simulink model "exampleModel_bus_axi_lcls2"  (R2017b)
settings: Solver=VariableStepAuto  StartTime=0.0  StopTime=10e-5  RelTol=1e-3
PreLoadFcn:
  | setup
values from neighbouring files (symbols this model uses):
  axiClk = 156.25e6    (= 156250000)    [setup.m]    (also in setup_exampleModel_bus_axi_simulink.m; setup_exampleModel_bus_axi_simulink_lcls2.m; setup_lcls2_pcav.m; sysgen_signal.m)
  cav1p1_addr = 204    [setup_exampleModel_bus_axi_simulink.m]    (also in setup_exampleModel_bus_axi_simulink_lcls2.m; setup_lcls2_pcav.m; sysgen_signal.m)
  cav1p2_addr = cav1p1_addr * 2    (= 408)    [setup_exampleModel_bus_axi_simulink.m]    (also in setup_exampleModel_bus_axi_simulink_lcls2.m; setup_lcls2_pcav.m; sysgen_signal.m)
  cav2p1_addr = cav1p1_addr * 3    (= 612)    [setup_exampleModel_bus_axi_simulink.m]    (also in setup_exampleModel_bus_axi_simulink_lcls2.m; setup_lcls2_pcav.m; sysgen_signal.m)
  cav2p2_addr = cav1p1_addr * 4    (= 816)    [setup_exampleModel_bus_axi_simulink.m]    (also in setup_exampleModel_bus_axi_simulink_lcls2.m; setup_lcls2_pcav.m; sysgen_signal.m)
  Fadc = Fs/interleavedChannels    (= 29750000)    [setup.m]    (also in setup_exampleModel_bus_axi_simulink.m = 357000000; setup_exampleModel_bus_axi_simulink_lcls2.m = 351000000; setup_lcls2_pcav.m = 357000000; sysgen_signal.m = 357000000)
  Fproc = 204e6    (= 204000000)    [setup_exampleModel_bus_axi_simulink.m]    (also in setup_exampleModel_bus_axi_simulink_lcls2.m = 200571400; setup_lcls2_pcav.m; sysgen_signal.m)
  Fsig = Fproc/12    (= 17000000)    [setup_exampleModel_bus_axi_simulink.m]    (also in setup_exampleModel_bus_axi_simulink_lcls2.m = 16714283.3333; setup_lcls2_pcav.m)
  Tadc = 1/fadc    (= 2.80112044818e-09)    [cavity_signal.m]    (also in setup_exampleModel_bus_axi_simulink.m; setup_exampleModel_bus_axi_simulink_lcls2.m = 2.849002849e-09; setup_lcls2_pcav.m; setup_pcav_simulink.m)
undefined symbols (not defined in the file or in its folder): AXI4, Lite
libraries: xbsIndex_r4 x2055, llrf_lib x10, simulink x1
(part 8 of 12)

== system exampleModel_bus_axi_lcls2/example/dsp/Cav2/c1p1_Masking_window ==
  note: delay for the comparison because Axilite register
      | takes a about 40 dsp clk cycles to load in
  counter : Inport
  start_pt : Inport  Port=2
  stop_pt : Inport  Port=3
  Constant1 : xbsIndex_r4/Constant  const=0  gui_display_data_type=Fixed-point  arith_type=Unsigned  n_bits=16  bin_pt=0  preci_type=Single  exp_width=8  frac_width=24  explicit_period=off  period=1  equ=P=C  opselect=C  inp2=PCIN>>17  opr=+  inp1=P  carry=CIN  dbl_ovrd=off  block_type=constant
  Convert11 : xbsIndex_r4/Convert  gui_display_data_type=Fixed-point  arith_type=Unsigned  n_bits=1  bin_pt=0  float_type=Single  exp_bits=8  fraction_bits=24  quantization=Truncate  overflow=Wrap  en=off  latency=1  pipeline=off  dbl_ovrd=off  block_type=convert
  Delay{1..4} (4 alike) : xbsIndex_r4/Delay  rst=off  infoeditControl=Selection of Reset will increase slice count due to use of real FFs and instead of SRLs  en=off  latency=1  reg_retiming=off  dbl_ovrd=off  block_type=delay
  Down Sample1 : xbsIndex_r4/Down Sample  sample_ratio=12  sample_phase="Last Value of Frame  (most efficient)"  en=off  rst=off  latency=1  dbl_ovrd=off  block_type=dsamp
  Down Sample2 : xbsIndex_r4/Down Sample  sample_ratio=12  sample_phase="Last Value of Frame  (most efficient)"  en=off  rst=off  latency=1  dbl_ovrd=off  block_type=dsamp
  Logical1 : xbsIndex_r4/Logical  logical_function=AND  inputs=2  en=off  latency=1  precision=Full  arith_type=Unsigned  n_bits=16  bin_pt=0  align_bp=on  dbl_ovrd=off  block_type=logical
  Register5 : xbsIndex_r4/Register  init=0  rst=off  en=off  dbl_ovrd=off  block_type=register
  Register6 : xbsIndex_r4/Register  init=100  rst=off  en=off  dbl_ovrd=off  block_type=register
  Relational2 : xbsIndex_r4/Relational  mode=a>b  op_type=Bool  en=off  latency=1  dbl_ovrd=off  block_type=relational
  Relational3 : xbsIndex_r4/Relational  mode=a<b  op_type=Bool  en=on  latency=1  dbl_ovrd=off  block_type=relational
  Relational4 : xbsIndex_r4/Relational  mode=a>b  op_type=Bool  en=on  latency=1  dbl_ovrd=off  block_type=relational
  eval_window : Outport
  wires:
  start_pt/1 -> Register5/1
  Register5/1 -> Down Sample1/1
  stop_pt/1 -> Register6/1
  Register6/1 -> Down Sample2/1
  Delay2/1 -> Relational4/2
  Delay3/1 -> [stop], Relational3/2
  Constant1/1 -> Relational2/2
  Logical1/1 -> Convert11/1
  Relational3/1 -> Logical1/2
  Convert11/1 -> eval_window/1
  Relational2/1 -> [enb], Relational3/3, Relational4/3
  counter/1 -> [cntr]
  Down Sample1/1 -> Delay2/1
  Down Sample2/1 -> Delay3/1
  Delay1/1 -> Relational4/1
  Delay4/1 -> Relational3/1
  Relational4/1 -> Logical1/1
  [cntr] -> Relational2/1, Delay1/1, Delay4/1

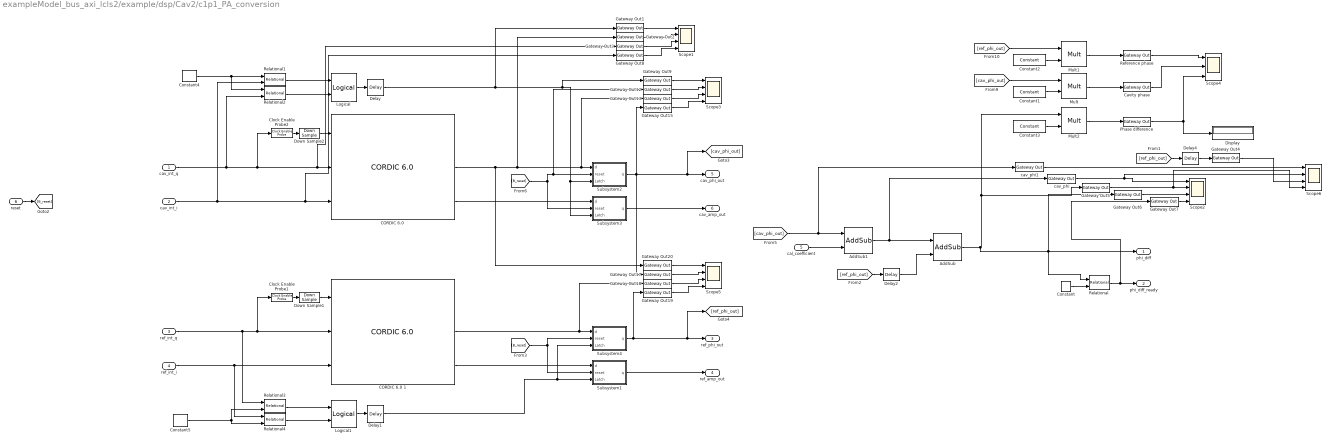
== system exampleModel_bus_axi_lcls2/example/dsp/Cav2/c1p1_PA_conversion ==
  cav_int_q : Inport
  cav_int_i : Inport  Port=2
  ref_int_q : Inport  Port=3
  ref_int_i : Inport  Port=4
  cal_coefficient : Inport  Port=5
  reset : Inport  Port=6
  AddSub : xbsIndex_r4/AddSub  mode=Subtraction  use_carryin=off  use_carryout=off  en=off  latency=1  precision=User Defined  arith_type="Signed  (2's comp)"  n_bits=18  bin_pt=15  quantization=Truncate  overflow=Wrap  use_behavioral_HDL=off  hw_selection=Fabric  pipelined=off  dbl_ovrd=off  block_type=addsub
  AddSub1 : xbsIndex_r4/AddSub  mode=Addition  use_carryin=off  use_carryout=off  en=off  latency=1  precision=User Defined  arith_type="Signed  (2's comp)"  n_bits=18  bin_pt=15  quantization=Truncate  overflow=Wrap  use_behavioral_HDL=off  hw_selection=Fabric  pipelined=off  dbl_ovrd=off  block_type=addsub
  "CORDIC 6.0 " : xbsIndex_r4/CORDIC 6.0   functional_selection=Translate  architectural_configuration=Parallel  pipelining_mode=Maximum  data_format=SignedFraction  phase_format=Scaled_Radians  input_width=18  output_width=18  round_mode=Truncate  iterations=0  precision=0  compensation_scaling=No_Scale_Compensation  coarse_rotation=on  aclken=off  aresetn=off  out_tready=off  cartesian_has_tuser=off  cartesian_has_tlast=off  cartesian_tuser_width=1  phase_has_tuser=off  phase_has_tlast=off  phase_tuser_width=1  out_tlast_behv=Null  flow_control=NonBlocking  optimize_goal=Resources  trim_axipin_name=on  simulation_type=hybrid_sim  simulation_model=sysgen:cordic_v6_0  data_path_portlist={'s_axis_cartesian_tdata_imag', 's_axis_cartesian_tdata_real', 's_axis_phase_tdata_phase', 'm_axis_dout_tdata_imag', 'm_axis_dout_tdata_real', 'm_axis_dout_tdata_phase','m_axis_dout_tdata'}  ip_name=CORDIC  ip_version=6.0  dsptool_ready=true  ipcore_usecache=true  ipcore_useipmodelcache=true  wrapper_available=true  port_translation_map={ 'aclken' => 'en', 'aresetn' => 'rst' }  block_type=cordic_v6_0
      settings: infoedit=CORDIC 6.0
  CORDIC 6.0 1 : xbsIndex_r4/CORDIC 6.0   functional_selection=Translate  architectural_configuration=Parallel  pipelining_mode=Maximum  data_format=SignedFraction  phase_format=Scaled_Radians  input_width=18  output_width=18  round_mode=Truncate  iterations=0  precision=0  compensation_scaling=No_Scale_Compensation  coarse_rotation=on  aclken=off  aresetn=off  out_tready=off  cartesian_has_tuser=off  cartesian_has_tlast=off  cartesian_tuser_width=1  phase_has_tuser=off  phase_has_tlast=off  phase_tuser_width=1  out_tlast_behv=Null  flow_control=NonBlocking  optimize_goal=Resources  trim_axipin_name=on  simulation_type=hybrid_sim  simulation_model=sysgen:cordic_v6_0  data_path_portlist={'s_axis_cartesian_tdata_imag', 's_axis_cartesian_tdata_real', 's_axis_phase_tdata_phase', 'm_axis_dout_tdata_imag', 'm_axis_dout_tdata_real', 'm_axis_dout_tdata_phase','m_axis_dout_tdata'}  ip_name=CORDIC  ip_version=6.0  dsptool_ready=true  ipcore_usecache=true  ipcore_useipmodelcache=true  wrapper_available=true  port_translation_map={ 'aclken' => 'en', 'aresetn' => 'rst' }  block_type=cordic_v6_0
      settings: infoedit=CORDIC 6.0
  Cavity phase : xbsIndex_r4/Gateway Out  inherit_from_input=off  hdl_port=off  rows=1  columns=1  UseAsDAC=off  DACChannel='1'  interface=None  automatic_assignment=on  address_offset=hex2dec('00')  intf_name=''  intf_description=''  timing_constraint=None  locs_specified=off  LOCs={}  io_standard={}  block_type=gatewayout
  Clock Enable Probe1 : xbsIndex_r4/Clock Enable Probe  inherit_constraints=on  block_type=ceprobe
      settings: infoedit="Clock enable extractor.  Produces a Boolean output that mirrors the hardware clock enable associated with the input sample rate.<br><br>Hardware notes: in hardware this block costs nothing."
  Clock Enable Probe2 : xbsIndex_r4/Clock Enable Probe  inherit_constraints=on  block_type=ceprobe
      settings: infoedit="Clock enable extractor.  Produces a Boolean output that mirrors the hardware clock enable associated with the input sample rate.<br><br>Hardware notes: in hardware this block costs nothing."
  Constant : xbsIndex_r4/Constant  const=0  gui_display_data_type=Fixed-point  arith_type=Signed (2's comp)  n_bits=1  bin_pt=0  preci_type=Single  exp_width=8  frac_width=24  explicit_period=off  period=1  equ=P=C  opselect=C  inp2=PCIN>>17  opr=+  inp1=P  carry=CIN  dbl_ovrd=off  block_type=constant
  Constant1 : xbsIndex_r4/Constant  const=pi  gui_display_data_type=Fixed-point  arith_type=Unsigned  n_bits=16  bin_pt=14  preci_type=Single  exp_width=8  frac_width=24  explicit_period=off  period=1  equ=P=C  opselect=C  inp2=PCIN>>17  opr=+  inp1=P  carry=CIN  dbl_ovrd=off  block_type=constant
  Constant2 : xbsIndex_r4/Constant  const=pi  gui_display_data_type=Fixed-point  arith_type=Unsigned  n_bits=16  bin_pt=14  preci_type=Single  exp_width=8  frac_width=24  explicit_period=off  period=1  equ=P=C  opselect=C  inp2=PCIN>>17  opr=+  inp1=P  carry=CIN  dbl_ovrd=off  block_type=constant
  Constant3 : xbsIndex_r4/Constant  const=pi  gui_display_data_type=Fixed-point  arith_type=Unsigned  n_bits=16  bin_pt=14  preci_type=Single  exp_width=8  frac_width=24  explicit_period=off  period=1  equ=P=C  opselect=C  inp2=PCIN>>17  opr=+  inp1=P  carry=CIN  dbl_ovrd=off  block_type=constant
  Constant4 : xbsIndex_r4/Constant  const=0  gui_display_data_type=Fixed-point  arith_type=Signed (2's comp)  n_bits=16  bin_pt=14  preci_type=Single  exp_width=8  frac_width=24  explicit_period=off  period=1  equ=P=C  opselect=C  inp2=PCIN>>17  opr=+  inp1=P  carry=CIN  dbl_ovrd=off  block_type=constant
  Constant5 : xbsIndex_r4/Constant  const=0  gui_display_data_type=Fixed-point  arith_type=Signed (2's comp)  n_bits=16  bin_pt=14  preci_type=Single  exp_width=8  frac_width=24  explicit_period=off  period=1  equ=P=C  opselect=C  inp2=PCIN>>17  opr=+  inp1=P  carry=CIN  dbl_ovrd=off  block_type=constant
  Delay : xbsIndex_r4/Delay  rst=off  infoeditControl=Selection of Reset will increase slice count due to use of real FFs and instead of SRLs  en=off  latency=21  reg_retiming=off  dbl_ovrd=off  block_type=delay
  Delay1 : xbsIndex_r4/Delay  rst=off  infoeditControl=Selection of Reset will increase slice count due to use of real FFs and instead of SRLs  en=off  latency=21  reg_retiming=off  dbl_ovrd=off  block_type=delay
  Delay2 : xbsIndex_r4/Delay  rst=off  infoeditControl=Selection of Reset will increase slice count due to use of real FFs and instead of SRLs  en=off  latency=1  reg_retiming=off  dbl_ovrd=off  block_type=delay
  Delay4 : xbsIndex_r4/Delay  rst=off  infoeditControl=Selection of Reset will increase slice count due to use of real FFs and instead of SRLs  en=off  latency=1  reg_retiming=off  dbl_ovrd=off  block_type=delay
  Display : Display
  Down Sample1 : xbsIndex_r4/Down Sample  sample_ratio=12  sample_phase="Last Value of Frame  (most efficient)"  en=off  rst=off  latency=1  dbl_ovrd=off  block_type=dsamp
  Down Sample2 : xbsIndex_r4/Down Sample  sample_ratio=12  sample_phase="Last Value of Frame  (most efficient)"  en=off  rst=off  latency=1  dbl_ovrd=off  block_type=dsamp
  Gateway Out{1..9,12..13,15,17..20} (16 alike) : xbsIndex_r4/Gateway Out  inherit_from_input=off  hdl_port=off  rows=1  columns=1  UseAsDAC=off  DACChannel='1'  interface=None  automatic_assignment=on  address_offset=hex2dec('00')  intf_name=''  intf_description=''  timing_constraint=None  locs_specified=off  LOCs={}  io_standard={}  block_type=gatewayout
  Logical : xbsIndex_r4/Logical  logical_function=AND  inputs=2  en=off  latency=1  precision=Full  arith_type=Unsigned  n_bits=16  bin_pt=0  align_bp=on  dbl_ovrd=off  block_type=logical
  Logical1 : xbsIndex_r4/Logical  logical_function=AND  inputs=2  en=off  latency=1  precision=Full  arith_type=Unsigned  n_bits=16  bin_pt=0  align_bp=on  dbl_ovrd=off  block_type=logical
  Mult : xbsIndex_r4/Mult  precision=Full  arith_type="Signed  (2's comp)"  n_bits=16  bin_pt=14  quantization=Truncate  overflow=Wrap  en=off  latency=3  use_behavioral_HDL=off  opt=Speed  use_embedded=on  optimum_pipeline=off  pipeline=on  dbl_ovrd=off  use_rpm=on  placement_style=Triangular  block_type=mult
  Mult1 : xbsIndex_r4/Mult  precision=Full  arith_type="Signed  (2's comp)"  n_bits=16  bin_pt=14  quantization=Truncate  overflow=Wrap  en=off  latency=3  use_behavioral_HDL=off  opt=Speed  use_embedded=on  optimum_pipeline=off  pipeline=on  dbl_ovrd=off  use_rpm=on  placement_style=Triangular  block_type=mult
  Mult2 : xbsIndex_r4/Mult  precision=Full  arith_type="Signed  (2's comp)"  n_bits=16  bin_pt=14  quantization=Truncate  overflow=Wrap  en=off  latency=3  use_behavioral_HDL=off  opt=Speed  use_embedded=on  optimum_pipeline=off  pipeline=on  dbl_ovrd=off  use_rpm=on  placement_style=Triangular  block_type=mult
  Phase difference : xbsIndex_r4/Gateway Out  inherit_from_input=off  hdl_port=off  rows=1  columns=1  UseAsDAC=off  DACChannel='1'  interface=None  automatic_assignment=on  address_offset=hex2dec('00')  intf_name=''  intf_description=''  timing_constraint=None  locs_specified=off  LOCs={}  io_standard={}  block_type=gatewayout
  Reference phase : xbsIndex_r4/Gateway Out  inherit_from_input=off  hdl_port=off  rows=1  columns=1  UseAsDAC=off  DACChannel='1'  interface=None  automatic_assignment=on  address_offset=hex2dec('00')  intf_name=''  intf_description=''  timing_constraint=None  locs_specified=off  LOCs={}  io_standard={}  block_type=gatewayout
  Relational{,1..4} (5 alike) : xbsIndex_r4/Relational  mode=a!=b  op_type=Bool  en=off  latency=1  dbl_ovrd=off  block_type=relational
  Scope{1..3,5..6} (5 alike) : Scope  NumInputPorts=4
  Scope4 : Scope  NumInputPorts=3
  Subsystem1 : Subsystem
  Subsystem2 : Subsystem
  Subsystem3 : Subsystem
  Subsystem4 : Subsystem
  cav_phi : xbsIndex_r4/Gateway Out  inherit_from_input=off  hdl_port=off  rows=1  columns=1  UseAsDAC=off  DACChannel='1'  interface=None  automatic_assignment=on  address_offset=hex2dec('00')  intf_name=''  intf_description=''  timing_constraint=None  locs_specified=off  LOCs={}  io_standard={}  block_type=gatewayout
  cav_phi1 : xbsIndex_r4/Gateway Out  inherit_from_input=off  hdl_port=off  rows=1  columns=1  UseAsDAC=off  DACChannel='1'  interface=None  automatic_assignment=on  address_offset=hex2dec('00')  intf_name=''  intf_description=''  timing_constraint=None  locs_specified=off  LOCs={}  io_standard={}  block_type=gatewayout
  phi_diff : Outport
  phi_diff_ready : Outport  Port=2
  ref_phi_out : Outport  Port=3
  ref_amp_out : Outport  Port=4
  cav_phi_out : Outport  Port=5
  cav_amp_out : Outport  Port=6
  wires:
  ref_int_i/1 -> CORDIC 6.0 1/3, Relational4/1
  ref_int_q/1 -> Relational3/1, CORDIC 6.0 1/2, Clock Enable Probe1/1
  [ref_phi_out] -> Delay4/1
  AddSub1/1 -> cav_phi/1, AddSub/1
  [cav_phi_out] -> cav_phi1/1, AddSub1/1
  cal_coefficient/1 -> AddSub1/2
  Subsystem4/1(q) -> Gateway Out19/1, [ref_phi_out], ref_phi_out/1
  Subsystem1/1(q) -> ref_amp_out/1
  Subsystem2/1(q) -> Gateway Out17/1, Gateway Out15/1, [cav_phi_out], cav_phi_out/1
  Subsystem3/1(q) -> cav_amp_out/1
  reset/1 -> [B_reset]
  [B_reset] -> Subsystem4/2(reset), Subsystem1/2(reset)
  [B_reset] -> Subsystem3/2(reset), Gateway Out12/1, Subsystem2/2(reset)
  AddSub/1 -> Gateway Out6/1, phi_diff/1, Relational/1, Mult2/1, Gateway Out5/1
  Delay2/1 -> AddSub/2
  Gateway Out5/1 -> Scope6/4, Scope2/2
  cav_phi/1 -> Scope6/2, Scope2/1
  Gateway Out6/1 -> Scope2/3
  Gateway Out7/1 -> Scope2/4
  Constant/1 -> Relational/2
  Relational/1 -> Gateway Out7/1, phi_diff_ready/1
  Constant1/1 -> Mult/2
  [cav_phi_out] -> Mult/1
  [ref_phi_out] -> Mult1/1
  Constant2/1 -> Mult1/2
  Mult1/1 -> Reference phase/1
  Mult/1 -> Cavity phase/1
  Mult2/1 -> Phase difference/1
  Constant3/1 -> Mult2/2
  Cavity phase/1 -> Scope4/2
  Reference phase/1 -> Scope4/1
  Phase difference/1 -> Display/1, Scope4/3
  Clock Enable Probe2/1 -> Down Sample2/1
  Down Sample2/1 -> "CORDIC 6.0 "/1
  cav_int_q/1 -> Relational2/2, Clock Enable Probe2/1, Gateway Out3/1, "CORDIC 6.0 "/2
  Logical/1 -> Delay/1
  Relational2/1 -> Logical/2
  Relational1/1 -> Logical/1
  cav_int_i/1 -> Relational1/2, Gateway Out8/1, "CORDIC 6.0 "/3
  Constant4/1 -> Relational2/1, Relational1/1
  Delay/1 -> Gateway Out1/1, Gateway Out9/1, Subsystem3/3(Latch), Subsystem2/3(Latch)
  Clock Enable Probe1/1 -> Down Sample1/1
  Down Sample1/1 -> CORDIC 6.0 1/1
  Delay1/1 -> Subsystem4/3(Latch), Subsystem1/3(Latch)
  Relational3/1 -> Logical1/1
  Relational4/1 -> Logical1/2
  Logical1/1 -> Delay1/1
  Constant5/1 -> Relational4/2, Relational3/2
  CORDIC 6.0 1/3 -> Subsystem1/1(d)
  CORDIC 6.0 1/2 -> Gateway Out18/1, Subsystem4/1(d)
  "CORDIC 6.0 "/2 -> Gateway Out20/1, Gateway Out2/1, Gateway Out13/1, Subsystem2/1(d)
  "CORDIC 6.0 "/3 -> Subsystem3/1(d)
  Gateway Out8/1 -> Scope1/4
  Gateway Out3/1 -> Scope1/3
  Gateway Out1/1 -> Scope1/1
  Gateway Out2/1 -> Scope1/2
  Gateway Out12/1 -> Scope3/2
  Gateway Out9/1 -> Scope3/1
  Gateway Out13/1 -> Scope3/3
  Gateway Out15/1 -> Scope3/4
  Gateway Out19/1 -> Scope5/4
  Gateway Out18/1 -> Scope5/3
  Gateway Out20/1 -> Scope5/1
  Gateway Out17/1 -> Scope5/2
  cav_phi1/1 -> Scope6/1
  Delay4/1 -> Gateway Out4/1
  Gateway Out4/1 -> Scope6/3
  [ref_phi_out] -> Delay2/1

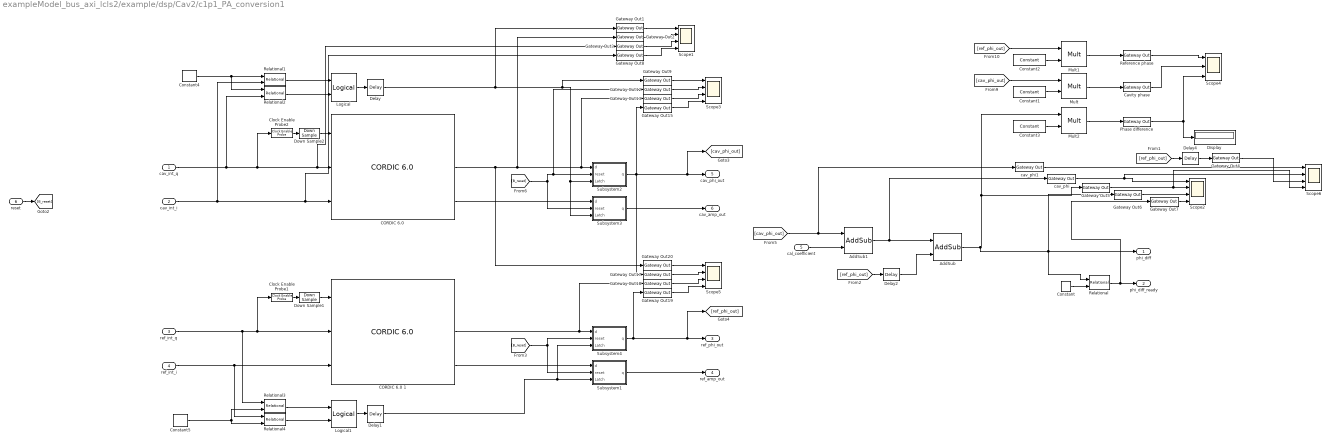
== system exampleModel_bus_axi_lcls2/example/dsp/Cav2/c1p1_PA_conversion1 ==
  cav_int_q : Inport
  cav_int_i : Inport  Port=2
  ref_int_q : Inport  Port=3
  ref_int_i : Inport  Port=4
  cal_coefficient : Inport  Port=5
  reset : Inport  Port=6
  AddSub : xbsIndex_r4/AddSub  mode=Subtraction  use_carryin=off  use_carryout=off  en=off  latency=1  precision=User Defined  arith_type="Signed  (2's comp)"  n_bits=18  bin_pt=15  quantization=Truncate  overflow=Wrap  use_behavioral_HDL=off  hw_selection=Fabric  pipelined=off  dbl_ovrd=off  block_type=addsub
  AddSub1 : xbsIndex_r4/AddSub  mode=Addition  use_carryin=off  use_carryout=off  en=off  latency=1  precision=User Defined  arith_type="Signed  (2's comp)"  n_bits=18  bin_pt=15  quantization=Truncate  overflow=Wrap  use_behavioral_HDL=off  hw_selection=Fabric  pipelined=off  dbl_ovrd=off  block_type=addsub
  "CORDIC 6.0 " : xbsIndex_r4/CORDIC 6.0   functional_selection=Translate  architectural_configuration=Parallel  pipelining_mode=Maximum  data_format=SignedFraction  phase_format=Scaled_Radians  input_width=18  output_width=18  round_mode=Truncate  iterations=0  precision=0  compensation_scaling=No_Scale_Compensation  coarse_rotation=on  aclken=off  aresetn=off  out_tready=off  cartesian_has_tuser=off  cartesian_has_tlast=off  cartesian_tuser_width=1  phase_has_tuser=off  phase_has_tlast=off  phase_tuser_width=1  out_tlast_behv=Null  flow_control=NonBlocking  optimize_goal=Resources  trim_axipin_name=on  simulation_type=hybrid_sim  simulation_model=sysgen:cordic_v6_0  data_path_portlist={'s_axis_cartesian_tdata_imag', 's_axis_cartesian_tdata_real', 's_axis_phase_tdata_phase', 'm_axis_dout_tdata_imag', 'm_axis_dout_tdata_real', 'm_axis_dout_tdata_phase','m_axis_dout_tdata'}  ip_name=CORDIC  ip_version=6.0  dsptool_ready=true  ipcore_usecache=true  ipcore_useipmodelcache=true  wrapper_available=true  port_translation_map={ 'aclken' => 'en', 'aresetn' => 'rst' }  block_type=cordic_v6_0
      settings: infoedit=CORDIC 6.0
  CORDIC 6.0 1 : xbsIndex_r4/CORDIC 6.0   functional_selection=Translate  architectural_configuration=Parallel  pipelining_mode=Maximum  data_format=SignedFraction  phase_format=Scaled_Radians  input_width=18  output_width=18  round_mode=Truncate  iterations=0  precision=0  compensation_scaling=No_Scale_Compensation  coarse_rotation=on  aclken=off  aresetn=off  out_tready=off  cartesian_has_tuser=off  cartesian_has_tlast=off  cartesian_tuser_width=1  phase_has_tuser=off  phase_has_tlast=off  phase_tuser_width=1  out_tlast_behv=Null  flow_control=NonBlocking  optimize_goal=Resources  trim_axipin_name=on  simulation_type=hybrid_sim  simulation_model=sysgen:cordic_v6_0  data_path_portlist={'s_axis_cartesian_tdata_imag', 's_axis_cartesian_tdata_real', 's_axis_phase_tdata_phase', 'm_axis_dout_tdata_imag', 'm_axis_dout_tdata_real', 'm_axis_dout_tdata_phase','m_axis_dout_tdata'}  ip_name=CORDIC  ip_version=6.0  dsptool_ready=true  ipcore_usecache=true  ipcore_useipmodelcache=true  wrapper_available=true  port_translation_map={ 'aclken' => 'en', 'aresetn' => 'rst' }  block_type=cordic_v6_0
      settings: infoedit=CORDIC 6.0
  Cavity phase : xbsIndex_r4/Gateway Out  inherit_from_input=off  hdl_port=off  rows=1  columns=1  UseAsDAC=off  DACChannel='1'  interface=None  automatic_assignment=on  address_offset=hex2dec('00')  intf_name=''  intf_description=''  timing_constraint=None  locs_specified=off  LOCs={}  io_standard={}  block_type=gatewayout
  Clock Enable Probe1 : xbsIndex_r4/Clock Enable Probe  inherit_constraints=on  block_type=ceprobe
      settings: infoedit="Clock enable extractor.  Produces a Boolean output that mirrors the hardware clock enable associated with the input sample rate.<br><br>Hardware notes: in hardware this block costs nothing."
  Clock Enable Probe2 : xbsIndex_r4/Clock Enable Probe  inherit_constraints=on  block_type=ceprobe
      settings: infoedit="Clock enable extractor.  Produces a Boolean output that mirrors the hardware clock enable associated with the input sample rate.<br><br>Hardware notes: in hardware this block costs nothing."
  Constant : xbsIndex_r4/Constant  const=0  gui_display_data_type=Fixed-point  arith_type=Signed (2's comp)  n_bits=1  bin_pt=0  preci_type=Single  exp_width=8  frac_width=24  explicit_period=off  period=1  equ=P=C  opselect=C  inp2=PCIN>>17  opr=+  inp1=P  carry=CIN  dbl_ovrd=off  block_type=constant
  Constant1 : xbsIndex_r4/Constant  const=pi  gui_display_data_type=Fixed-point  arith_type=Unsigned  n_bits=16  bin_pt=14  preci_type=Single  exp_width=8  frac_width=24  explicit_period=off  period=1  equ=P=C  opselect=C  inp2=PCIN>>17  opr=+  inp1=P  carry=CIN  dbl_ovrd=off  block_type=constant
  Constant2 : xbsIndex_r4/Constant  const=pi  gui_display_data_type=Fixed-point  arith_type=Unsigned  n_bits=16  bin_pt=14  preci_type=Single  exp_width=8  frac_width=24  explicit_period=off  period=1  equ=P=C  opselect=C  inp2=PCIN>>17  opr=+  inp1=P  carry=CIN  dbl_ovrd=off  block_type=constant
  Constant3 : xbsIndex_r4/Constant  const=pi  gui_display_data_type=Fixed-point  arith_type=Unsigned  n_bits=16  bin_pt=14  preci_type=Single  exp_width=8  frac_width=24  explicit_period=off  period=1  equ=P=C  opselect=C  inp2=PCIN>>17  opr=+  inp1=P  carry=CIN  dbl_ovrd=off  block_type=constant
  Constant4 : xbsIndex_r4/Constant  const=0  gui_display_data_type=Fixed-point  arith_type=Signed (2's comp)  n_bits=16  bin_pt=14  preci_type=Single  exp_width=8  frac_width=24  explicit_period=off  period=1  equ=P=C  opselect=C  inp2=PCIN>>17  opr=+  inp1=P  carry=CIN  dbl_ovrd=off  block_type=constant
  Constant5 : xbsIndex_r4/Constant  const=0  gui_display_data_type=Fixed-point  arith_type=Signed (2's comp)  n_bits=16  bin_pt=14  preci_type=Single  exp_width=8  frac_width=24  explicit_period=off  period=1  equ=P=C  opselect=C  inp2=PCIN>>17  opr=+  inp1=P  carry=CIN  dbl_ovrd=off  block_type=constant
  Delay : xbsIndex_r4/Delay  rst=off  infoeditControl=Selection of Reset will increase slice count due to use of real FFs and instead of SRLs  en=off  latency=21  reg_retiming=off  dbl_ovrd=off  block_type=delay
  Delay1 : xbsIndex_r4/Delay  rst=off  infoeditControl=Selection of Reset will increase slice count due to use of real FFs and instead of SRLs  en=off  latency=21  reg_retiming=off  dbl_ovrd=off  block_type=delay
  Delay2 : xbsIndex_r4/Delay  rst=off  infoeditControl=Selection of Reset will increase slice count due to use of real FFs and instead of SRLs  en=off  latency=1  reg_retiming=off  dbl_ovrd=off  block_type=delay
  Delay4 : xbsIndex_r4/Delay  rst=off  infoeditControl=Selection of Reset will increase slice count due to use of real FFs and instead of SRLs  en=off  latency=1  reg_retiming=off  dbl_ovrd=off  block_type=delay
  Display : Display
  Down Sample1 : xbsIndex_r4/Down Sample  sample_ratio=12  sample_phase="Last Value of Frame  (most efficient)"  en=off  rst=off  latency=1  dbl_ovrd=off  block_type=dsamp
  Down Sample2 : xbsIndex_r4/Down Sample  sample_ratio=12  sample_phase="Last Value of Frame  (most efficient)"  en=off  rst=off  latency=1  dbl_ovrd=off  block_type=dsamp
  Gateway Out{1..9,12..13,15,17..20} (16 alike) : xbsIndex_r4/Gateway Out  inherit_from_input=off  hdl_port=off  rows=1  columns=1  UseAsDAC=off  DACChannel='1'  interface=None  automatic_assignment=on  address_offset=hex2dec('00')  intf_name=''  intf_description=''  timing_constraint=None  locs_specified=off  LOCs={}  io_standard={}  block_type=gatewayout
  Logical : xbsIndex_r4/Logical  logical_function=AND  inputs=2  en=off  latency=1  precision=Full  arith_type=Unsigned  n_bits=16  bin_pt=0  align_bp=on  dbl_ovrd=off  block_type=logical
  Logical1 : xbsIndex_r4/Logical  logical_function=AND  inputs=2  en=off  latency=1  precision=Full  arith_type=Unsigned  n_bits=16  bin_pt=0  align_bp=on  dbl_ovrd=off  block_type=logical
  Mult : xbsIndex_r4/Mult  precision=Full  arith_type="Signed  (2's comp)"  n_bits=16  bin_pt=14  quantization=Truncate  overflow=Wrap  en=off  latency=3  use_behavioral_HDL=off  opt=Speed  use_embedded=on  optimum_pipeline=off  pipeline=on  dbl_ovrd=off  use_rpm=on  placement_style=Triangular  block_type=mult
  Mult1 : xbsIndex_r4/Mult  precision=Full  arith_type="Signed  (2's comp)"  n_bits=16  bin_pt=14  quantization=Truncate  overflow=Wrap  en=off  latency=3  use_behavioral_HDL=off  opt=Speed  use_embedded=on  optimum_pipeline=off  pipeline=on  dbl_ovrd=off  use_rpm=on  placement_style=Triangular  block_type=mult
  Mult2 : xbsIndex_r4/Mult  precision=Full  arith_type="Signed  (2's comp)"  n_bits=16  bin_pt=14  quantization=Truncate  overflow=Wrap  en=off  latency=3  use_behavioral_HDL=off  opt=Speed  use_embedded=on  optimum_pipeline=off  pipeline=on  dbl_ovrd=off  use_rpm=on  placement_style=Triangular  block_type=mult
  Phase difference : xbsIndex_r4/Gateway Out  inherit_from_input=off  hdl_port=off  rows=1  columns=1  UseAsDAC=off  DACChannel='1'  interface=None  automatic_assignment=on  address_offset=hex2dec('00')  intf_name=''  intf_description=''  timing_constraint=None  locs_specified=off  LOCs={}  io_standard={}  block_type=gatewayout
  Reference phase : xbsIndex_r4/Gateway Out  inherit_from_input=off  hdl_port=off  rows=1  columns=1  UseAsDAC=off  DACChannel='1'  interface=None  automatic_assignment=on  address_offset=hex2dec('00')  intf_name=''  intf_description=''  timing_constraint=None  locs_specified=off  LOCs={}  io_standard={}  block_type=gatewayout
  Relational{,1..4} (5 alike) : xbsIndex_r4/Relational  mode=a!=b  op_type=Bool  en=off  latency=1  dbl_ovrd=off  block_type=relational
  Scope{1..3,5..6} (5 alike) : Scope  NumInputPorts=4
  Scope4 : Scope  NumInputPorts=3
  Subsystem1 : Subsystem
  Subsystem2 : Subsystem
  Subsystem3 : Subsystem
  Subsystem4 : Subsystem
  cav_phi : xbsIndex_r4/Gateway Out  inherit_from_input=off  hdl_port=off  rows=1  columns=1  UseAsDAC=off  DACChannel='1'  interface=None  automatic_assignment=on  address_offset=hex2dec('00')  intf_name=''  intf_description=''  timing_constraint=None  locs_specified=off  LOCs={}  io_standard={}  block_type=gatewayout
  cav_phi1 : xbsIndex_r4/Gateway Out  inherit_from_input=off  hdl_port=off  rows=1  columns=1  UseAsDAC=off  DACChannel='1'  interface=None  automatic_assignment=on  address_offset=hex2dec('00')  intf_name=''  intf_description=''  timing_constraint=None  locs_specified=off  LOCs={}  io_standard={}  block_type=gatewayout
  phi_diff : Outport
  phi_diff_ready : Outport  Port=2
  ref_phi_out : Outport  Port=3
  ref_amp_out : Outport  Port=4
  cav_phi_out : Outport  Port=5
  cav_amp_out : Outport  Port=6
  wires:
  ref_int_i/1 -> CORDIC 6.0 1/3, Relational4/1
  ref_int_q/1 -> Relational3/1, CORDIC 6.0 1/2, Clock Enable Probe1/1
  [ref_phi_out] -> Delay4/1
  AddSub1/1 -> cav_phi/1, AddSub/1
  [cav_phi_out] -> cav_phi1/1, AddSub1/1
  cal_coefficient/1 -> AddSub1/2
  Subsystem4/1(q) -> Gateway Out19/1, [ref_phi_out], ref_phi_out/1
  Subsystem1/1(q) -> ref_amp_out/1
  Subsystem2/1(q) -> Gateway Out17/1, Gateway Out15/1, [cav_phi_out], cav_phi_out/1
  Subsystem3/1(q) -> cav_amp_out/1
  reset/1 -> [B_reset]
  [B_reset] -> Subsystem4/2(reset), Subsystem1/2(reset)
  [B_reset] -> Subsystem3/2(reset), Gateway Out12/1, Subsystem2/2(reset)
  AddSub/1 -> Gateway Out6/1, phi_diff/1, Relational/1, Mult2/1, Gateway Out5/1
  Delay2/1 -> AddSub/2
  Gateway Out5/1 -> Scope6/4, Scope2/2
  cav_phi/1 -> Scope6/2, Scope2/1
  Gateway Out6/1 -> Scope2/3
  Gateway Out7/1 -> Scope2/4
  Constant/1 -> Relational/2
  Relational/1 -> Gateway Out7/1, phi_diff_ready/1
  Constant1/1 -> Mult/2
  [cav_phi_out] -> Mult/1
  [ref_phi_out] -> Mult1/1
  Constant2/1 -> Mult1/2
  Mult1/1 -> Reference phase/1
  Mult/1 -> Cavity phase/1
  Mult2/1 -> Phase difference/1
  Constant3/1 -> Mult2/2
  Cavity phase/1 -> Scope4/2
  Reference phase/1 -> Scope4/1
  Phase difference/1 -> Display/1, Scope4/3
  Clock Enable Probe2/1 -> Down Sample2/1
  Down Sample2/1 -> "CORDIC 6.0 "/1
  cav_int_q/1 -> Relational2/2, Clock Enable Probe2/1, Gateway Out3/1, "CORDIC 6.0 "/2
  Logical/1 -> Delay/1
  Relational2/1 -> Logical/2
  Relational1/1 -> Logical/1
  cav_int_i/1 -> Relational1/2, Gateway Out8/1, "CORDIC 6.0 "/3
  Constant4/1 -> Relational2/1, Relational1/1
  Delay/1 -> Gateway Out1/1, Gateway Out9/1, Subsystem3/3(Latch), Subsystem2/3(Latch)
  Clock Enable Probe1/1 -> Down Sample1/1
  Down Sample1/1 -> CORDIC 6.0 1/1
  Delay1/1 -> Subsystem4/3(Latch), Subsystem1/3(Latch)
  Relational3/1 -> Logical1/1
  Relational4/1 -> Logical1/2
  Logical1/1 -> Delay1/1
  Constant5/1 -> Relational4/2, Relational3/2
  CORDIC 6.0 1/3 -> Subsystem1/1(d)
  CORDIC 6.0 1/2 -> Gateway Out18/1, Subsystem4/1(d)
  "CORDIC 6.0 "/2 -> Gateway Out20/1, Gateway Out2/1, Gateway Out13/1, Subsystem2/1(d)
  "CORDIC 6.0 "/3 -> Subsystem3/1(d)
  Gateway Out8/1 -> Scope1/4
  Gateway Out3/1 -> Scope1/3
  Gateway Out1/1 -> Scope1/1
  Gateway Out2/1 -> Scope1/2
  Gateway Out12/1 -> Scope3/2
  Gateway Out9/1 -> Scope3/1
  Gateway Out13/1 -> Scope3/3
  Gateway Out15/1 -> Scope3/4
  Gateway Out19/1 -> Scope5/4
  Gateway Out18/1 -> Scope5/3
  Gateway Out20/1 -> Scope5/1
  Gateway Out17/1 -> Scope5/2
  cav_phi1/1 -> Scope6/1
  Delay4/1 -> Gateway Out4/1
  Gateway Out4/1 -> Scope6/3
  [ref_phi_out] -> Delay2/1

== system exampleModel_bus_axi_lcls2/example/dsp/Cav2/c1p2_freq_err_module1 ==
  imag : Inport
  real : Inport  Port=2
  flo_window : Inport  Port=3
  reset : Inport  Port=4
  CORDIC 6.0 2 : xbsIndex_r4/CORDIC 6.0   functional_selection=Translate  architectural_configuration=Parallel  pipelining_mode=Maximum  data_format=SignedFraction  phase_format=Radians  input_width=18  output_width=18  round_mode=Truncate  iterations=0  precision=0  compensation_scaling=No_Scale_Compensation  coarse_rotation=on  aclken=off  aresetn=off  out_tready=off  cartesian_has_tuser=off  cartesian_has_tlast=off  cartesian_tuser_width=1  phase_has_tuser=off  phase_has_tlast=off  phase_tuser_width=1  out_tlast_behv=Null  flow_control=NonBlocking  optimize_goal=Resources  trim_axipin_name=on  simulation_type=hybrid_sim  simulation_model=sysgen:cordic_v6_0  data_path_portlist={'s_axis_cartesian_tdata_imag', 's_axis_cartesian_tdata_real', 's_axis_phase_tdata_phase', 'm_axis_dout_tdata_imag', 'm_axis_dout_tdata_real', 'm_axis_dout_tdata_phase','m_axis_dout_tdata'}  ip_name=CORDIC  ip_version=6.0  dsptool_ready=true  ipcore_usecache=true  ipcore_useipmodelcache=true  wrapper_available=true  port_translation_map={ 'aclken' => 'en', 'aresetn' => 'rst' }  block_type=cordic_v6_0
      settings: infoedit=CORDIC 6.0
  Clock Enable Probe4 : xbsIndex_r4/Clock Enable Probe  inherit_constraints=on  block_type=ceprobe
      settings: infoedit="Clock enable extractor.  Produces a Boolean output that mirrors the hardware clock enable associated with the input sample rate.<br><br>Hardware notes: in hardware this block costs nothing."
  Down Sample5 : xbsIndex_r4/Down Sample  sample_ratio=12  sample_phase="Last Value of Frame  (most efficient)"  en=off  rst=off  latency=1  dbl_ovrd=off  block_type=dsamp
  Gateway Out{1..5,38,41,53} (8 alike) : xbsIndex_r4/Gateway Out  inherit_from_input=off  hdl_port=off  rows=1  columns=1  UseAsDAC=off  DACChannel='1'  interface=None  automatic_assignment=on  address_offset=hex2dec('00')  intf_name=''  intf_description=''  timing_constraint=None  locs_specified=off  LOCs={}  io_standard={}  block_type=gatewayout
  Gateway Out44 : xbsIndex_r4/Gateway Out  inherit_from_input=off  hdl_port=on  rows=1  columns=1  UseAsDAC=off  DACChannel='1'  interface=None  automatic_assignment=on  address_offset=hex2dec('00')  intf_name=''  intf_description=''  timing_constraint=None  locs_specified=off  LOCs={}  io_standard={}  block_type=gatewayout
  Gateway Out46 : xbsIndex_r4/Gateway Out  inherit_from_input=off  hdl_port=on  rows=1  columns=1  UseAsDAC=off  DACChannel='1'  interface=None  automatic_assignment=on  address_offset=hex2dec('00')  intf_name=''  intf_description=''  timing_constraint=None  locs_specified=off  LOCs={}  io_standard={}  block_type=gatewayout
  Mult3 : xbsIndex_r4/Mult  precision=User Defined  arith_type="Signed  (2's comp)"  n_bits=18  bin_pt=15  quantization=Truncate  overflow=Saturate  en=off  latency=3  use_behavioral_HDL=off  opt=Speed  use_embedded=on  optimum_pipeline=off  pipeline=on  dbl_ovrd=off  use_rpm=on  placement_style=Triangular  block_type=mult
  Scope1 : Scope  NumInputPorts=4
  Scope21 : Scope  NumInputPorts=4
  Scope22 : Scope  NumInputPorts=2
  freq_err1 : Subsystem
  NCO_err_fb : Outport
  freq_err : Outport  Port=2
  tag scope: cav2_freq_phase=global
  wires:
  Gateway Out2/1 -> Scope1/4
  Gateway Out1/1 -> Scope1/3
  Gateway Out4/1 -> Scope1/1
  Gateway Out3/1 -> Scope1/2
  Mult3/1 -> Gateway Out1/1
  [cav1_pt_cntr] -> Gateway Out2/1
  freq_err1/2(freq_err) -> freq_err/1
  Gateway Out46/1 -> Scope22/1
  freq_err1/1(NCO_err) -> NCO_err_fb/1
  Gateway Out41/1 -> Scope21/3
  Gateway Out53/1 -> Scope21/1
  Gateway Out44/1 -> Scope22/2
  flo_window/1 -> freq_err1/2(window), Mult3/2, Gateway Out3/1
  imag/1 -> Gateway Out46/1, Clock Enable Probe4/1, CORDIC 6.0 2/2
  real/1 -> Gateway Out44/1, CORDIC 6.0 2/3
  CORDIC 6.0 2/2 -> Gateway Out38/1, [cav2_freq_phase], freq_err1/1(raw_phase)
  Clock Enable Probe4/1 -> Down Sample5/1
  CORDIC 6.0 2/3 -> Gateway Out53/1, Mult3/1, Gateway Out4/1
  reset/1 -> freq_err1/3(reset)
  Gateway Out38/1 -> Scope21/2
  Down Sample5/1 -> CORDIC 6.0 2/1
  [cav1_pt_cntr] -> Gateway Out41/1
  [c1p1_pt_window] -> Gateway Out5/1
  Gateway Out5/1 -> Scope21/4

== system exampleModel_bus_axi_lcls2/example/dsp/Cav2/c1p2_freq_err_module2 ==
  imag : Inport
  real : Inport  Port=2
  flo_window : Inport  Port=3
  reset : Inport  Port=4
  CORDIC 6.0 2 : xbsIndex_r4/CORDIC 6.0   functional_selection=Translate  architectural_configuration=Parallel  pipelining_mode=Maximum  data_format=SignedFraction  phase_format=Radians  input_width=18  output_width=18  round_mode=Truncate  iterations=0  precision=0  compensation_scaling=No_Scale_Compensation  coarse_rotation=on  aclken=off  aresetn=off  out_tready=off  cartesian_has_tuser=off  cartesian_has_tlast=off  cartesian_tuser_width=1  phase_has_tuser=off  phase_has_tlast=off  phase_tuser_width=1  out_tlast_behv=Null  flow_control=NonBlocking  optimize_goal=Resources  trim_axipin_name=on  simulation_type=hybrid_sim  simulation_model=sysgen:cordic_v6_0  data_path_portlist={'s_axis_cartesian_tdata_imag', 's_axis_cartesian_tdata_real', 's_axis_phase_tdata_phase', 'm_axis_dout_tdata_imag', 'm_axis_dout_tdata_real', 'm_axis_dout_tdata_phase','m_axis_dout_tdata'}  ip_name=CORDIC  ip_version=6.0  dsptool_ready=true  ipcore_usecache=true  ipcore_useipmodelcache=true  wrapper_available=true  port_translation_map={ 'aclken' => 'en', 'aresetn' => 'rst' }  block_type=cordic_v6_0
      settings: infoedit=CORDIC 6.0
  Clock Enable Probe4 : xbsIndex_r4/Clock Enable Probe  inherit_constraints=on  block_type=ceprobe
      settings: infoedit="Clock enable extractor.  Produces a Boolean output that mirrors the hardware clock enable associated with the input sample rate.<br><br>Hardware notes: in hardware this block costs nothing."
  Down Sample5 : xbsIndex_r4/Down Sample  sample_ratio=12  sample_phase="Last Value of Frame  (most efficient)"  en=off  rst=off  latency=1  dbl_ovrd=off  block_type=dsamp
  Gateway Out{1..5,38,41,53} (8 alike) : xbsIndex_r4/Gateway Out  inherit_from_input=off  hdl_port=off  rows=1  columns=1  UseAsDAC=off  DACChannel='1'  interface=None  automatic_assignment=on  address_offset=hex2dec('00')  intf_name=''  intf_description=''  timing_constraint=None  locs_specified=off  LOCs={}  io_standard={}  block_type=gatewayout
  Gateway Out44 : xbsIndex_r4/Gateway Out  inherit_from_input=off  hdl_port=on  rows=1  columns=1  UseAsDAC=off  DACChannel='1'  interface=None  automatic_assignment=on  address_offset=hex2dec('00')  intf_name=''  intf_description=''  timing_constraint=None  locs_specified=off  LOCs={}  io_standard={}  block_type=gatewayout
  Gateway Out46 : xbsIndex_r4/Gateway Out  inherit_from_input=off  hdl_port=on  rows=1  columns=1  UseAsDAC=off  DACChannel='1'  interface=None  automatic_assignment=on  address_offset=hex2dec('00')  intf_name=''  intf_description=''  timing_constraint=None  locs_specified=off  LOCs={}  io_standard={}  block_type=gatewayout
  Mult3 : xbsIndex_r4/Mult  precision=User Defined  arith_type="Signed  (2's comp)"  n_bits=18  bin_pt=15  quantization=Truncate  overflow=Saturate  en=off  latency=3  use_behavioral_HDL=off  opt=Speed  use_embedded=on  optimum_pipeline=off  pipeline=on  dbl_ovrd=off  use_rpm=on  placement_style=Triangular  block_type=mult
  Scope1 : Scope  NumInputPorts=4
  Scope21 : Scope  NumInputPorts=4
  Scope22 : Scope  NumInputPorts=2
  freq_err1 : Subsystem
  NCO_err_fb : Outport
  freq_err : Outport  Port=2
  tag scope: cav2_fll_amp_raw=global, cav2_fll_amp_windowed=global
  wires:
  Gateway Out2/1 -> Scope1/4
  Gateway Out1/1 -> Scope1/3
  Gateway Out4/1 -> Scope1/1
  Gateway Out3/1 -> Scope1/2
  Mult3/1 -> [cav2_fll_amp_windowed], Gateway Out1/1
  [cav1_pt_cntr] -> Gateway Out2/1
  freq_err1/2(freq_err) -> freq_err/1
  Gateway Out46/1 -> Scope22/1
  freq_err1/1(NCO_err) -> NCO_err_fb/1
  Gateway Out41/1 -> Scope21/3
  Gateway Out53/1 -> Scope21/1
  Gateway Out44/1 -> Scope22/2
  flo_window/1 -> freq_err1/2(window), Mult3/2, Gateway Out3/1
  imag/1 -> Gateway Out46/1, Clock Enable Probe4/1, CORDIC 6.0 2/2
  real/1 -> Gateway Out44/1, CORDIC 6.0 2/3
  CORDIC 6.0 2/2 -> Gateway Out38/1, freq_err1/1(raw_phase)
  Clock Enable Probe4/1 -> Down Sample5/1
  CORDIC 6.0 2/3 -> Gateway Out53/1, [cav2_fll_amp_raw], Mult3/1, Gateway Out4/1
  reset/1 -> freq_err1/3(reset)
  Gateway Out38/1 -> Scope21/2
  Down Sample5/1 -> CORDIC 6.0 2/1
  [cav1_pt_cntr] -> Gateway Out41/1
  [c1p1_pt_window] -> Gateway Out5/1
  Gateway Out5/1 -> Scope21/4

== system exampleModel_bus_axi_lcls2/example/dsp/Cav2/c1p2_window_wf ==
  cav_img : Inport
  cav_real : Inport  Port=2
  ref_img : Inport  Port=3
  ref_real : Inport  Port=4
  pt_window : Inport  Port=5
  Mult{,2,4..5} (4 alike) : xbsIndex_r4/Mult  precision=User Defined  arith_type="Signed  (2's comp)"  n_bits=18  bin_pt=16  quantization=Truncate  overflow=Wrap  en=off  latency=3  use_behavioral_HDL=off  opt=Speed  use_embedded=on  optimum_pipeline=off  pipeline=on  dbl_ovrd=off  use_rpm=on  placement_style=Triangular  block_type=mult
  cav_windowed_imag : Outport
  cav_windowed_real : Outport  Port=2
  ref_windowed_imag : Outport  Port=3
  ref_windowed_real : Outport  Port=4
  wires:
  Mult2/1 -> cav_windowed_imag/1
  [pt_win] -> Mult2/2
  Mult/1 -> cav_windowed_real/1
  [pt_win] -> Mult/2
  ref_img/1 -> Mult5/1
  [pt_win] -> Mult5/2
  [pt_win] -> Mult4/2
  ref_real/1 -> Mult4/1
  Mult5/1 -> ref_windowed_imag/1
  Mult4/1 -> ref_windowed_real/1
  pt_window/1 -> [pt_win]
  cav_real/1 -> Mult/1
  cav_img/1 -> Mult2/1

== system exampleModel_bus_axi_lcls2/example/dsp/Cav2/c2p1_window_wf  ==
  cav_img : Inport
  cav_real : Inport  Port=2
  ref_img : Inport  Port=3
  ref_real : Inport  Port=4
  pt_window : Inport  Port=5
  Mult{,2,4..5} (4 alike) : xbsIndex_r4/Mult  precision=User Defined  arith_type="Signed  (2's comp)"  n_bits=18  bin_pt=16  quantization=Truncate  overflow=Wrap  en=off  latency=3  use_behavioral_HDL=off  opt=Speed  use_embedded=on  optimum_pipeline=off  pipeline=on  dbl_ovrd=off  use_rpm=on  placement_style=Triangular  block_type=mult
  cav_windowed_imag : Outport
  cav_windowed_real : Outport  Port=2
  ref_windowed_imag : Outport  Port=3
  ref_windowed_real : Outport  Port=4
  wires:
  Mult2/1 -> cav_windowed_imag/1
  [pt_win] -> Mult2/2
  Mult/1 -> cav_windowed_real/1
  [pt_win] -> Mult/2
  ref_img/1 -> Mult5/1
  [pt_win] -> Mult5/2
  [pt_win] -> Mult4/2
  ref_real/1 -> Mult4/1
  Mult5/1 -> ref_windowed_imag/1
  Mult4/1 -> ref_windowed_real/1
  pt_window/1 -> [pt_win]
  cav_real/1 -> Mult/1
  cav_img/1 -> Mult2/1

== system exampleModel_bus_axi_lcls2/example/dsp/Ref/IQ_select ==
  IQ_stream_in : Inport
  IQ_chan_sel : Inport  Port=2
  Bus Creator5 : BusCreator  Inputs=3
  Bus Selector : BusSelector  OutputSignals=ddcI,ddcQ,sync
  Bus Selector3 : BusSelector  OutputSignals=ddcI,ddcQ,ddcSync,ddcChannel
  Channel Select3 : llrf_lib/Sysgen/Single Rate/Channel Select  SystemSampleTime=-1
      settings: SourceProductName=LLRF Library
  ddcI : Outport
  ddcQ : Outport  Port=2
  sync : Outport  Port=3
  wires:
  IQ_stream_in/1 -> Bus Selector3/1
  IQ_chan_sel/1 -> Channel Select3/5
  Channel Select3/3 -> Bus Creator5/3  "sync"
  Bus Selector3/2 -> Channel Select3/2  "<ddcQ>"
  Channel Select3/1 -> Bus Creator5/1  "ddcI"
  Channel Select3/2 -> Bus Creator5/2  "ddcQ"
  Bus Selector3/1 -> Channel Select3/1  "<ddcI>"
  Bus Selector3/4 -> Channel Select3/4  "<ddcChannel>"
  Bus Selector3/3 -> Channel Select3/3  "<ddcSync>"
  Bus Creator5/1 -> Bus Selector/1
  Bus Selector/1 -> ddcI/1  "<ddcI>"
  Bus Selector/2 -> ddcQ/1  "<ddcQ>"
  Bus Selector/3 -> sync/1  "<sync>"

== system exampleModel_bus_axi_lcls2/example/dsp/Ref/PA_select ==
  PA_bus : Inport
  PA_chan_sel : Inport  Port=2
  Bus Selector1 : BusSelector  OutputSignals=amp,phase,sync,channel
  Channel Select1 : llrf_lib/Sysgen/Single Rate/Channel Select  SystemSampleTime=-1
      settings: SourceProductName=LLRF Library
  Amp : Outport
  Phase : Outport  Port=2
  sync : Outport  Port=3
  wires:
  PA_bus/1 -> Bus Selector1/1
  PA_chan_sel/1 -> Channel Select1/5
  Channel Select1/3 -> sync/1  "sync"
  Channel Select1/2 -> Phase/1  "phase"
  Channel Select1/1 -> Amp/1  "amp"
  Bus Selector1/4 -> Channel Select1/4  "<channel>"
  Bus Selector1/3 -> Channel Select1/3  "<sync>"
  Bus Selector1/2 -> Channel Select1/2  "<phase>"
  Bus Selector1/1 -> Channel Select1/1  "<amp>"

== system exampleModel_bus_axi_lcls2/example/dsp/Cav1/DDC NCO1/pulse_catcher ==
  In1 : Inport
  Convert : xbsIndex_r4/Convert  gui_display_data_type=Boolean  arith_type=Boolean  n_bits=16  bin_pt=14  float_type=Single  exp_bits=8  fraction_bits=24  quantization=Truncate  overflow=Wrap  en=off  latency=1  pipeline=off  dbl_ovrd=off  block_type=convert
  Delay : xbsIndex_r4/Delay  rst=off  infoeditControl=Selection of Reset will increase slice count due to use of real FFs and instead of SRLs  en=off  latency=5  reg_retiming=off  dbl_ovrd=off  block_type=delay
  Delay1 : xbsIndex_r4/Delay  rst=off  infoeditControl=Selection of Reset will increase slice count due to use of real FFs and instead of SRLs  en=off  latency=1  reg_retiming=off  dbl_ovrd=off  block_type=delay
  Register : xbsIndex_r4/Register  init=0  rst=on  en=on  dbl_ovrd=off  block_type=register
  Out1 : Outport
  wires:
  In1/1 -> Convert/1, Delay1/1
  Delay/1 -> Register/2
  Register/1 -> Out1/1
  Convert/1 -> Register/3, Delay/1
  Delay1/1 -> Register/1

== system exampleModel_bus_axi_lcls2/example/dsp/Cav1/IQ_integration1/IQ_latch_normalize ==
  I : Inport
  Q : Inport  Port=2
  Window : Inport  Port=3
  Reset : Inport  Port=4
  Accumulator4 : xbsIndex_r4/Accumulator  operation=Add  n_bits=26  overflow=Wrap  scale=1  rst=on  hasbypass=off  infoeditControl=reset for floating point data type must be asserted for a minimum of 2 cycles  en=off  latency=1  msb_inp=100  msb=100  lsb=-100  use_behavioral_HDL=on  implementation=Fabric  dbl_ovrd=off  block_type=accum
  Accumulator5 : xbsIndex_r4/Accumulator  operation=Add  n_bits=26  overflow=Wrap  scale=1  rst=on  hasbypass=off  infoeditControl=reset for floating point data type must be asserted for a minimum of 2 cycles  en=off  latency=1  msb_inp=100  msb=100  lsb=-100  use_behavioral_HDL=on  implementation=Fabric  dbl_ovrd=off  block_type=accum
  Convert10 : xbsIndex_r4/Convert  gui_display_data_type=Boolean  arith_type=Boolean  n_bits=16  bin_pt=14  float_type=Single  exp_bits=8  fraction_bits=24  quantization=Truncate  overflow=Wrap  en=off  latency=1  pipeline=off  dbl_ovrd=off  block_type=convert
  Convert7 : xbsIndex_r4/Convert  gui_display_data_type=Boolean  arith_type=Boolean  n_bits=16  bin_pt=14  float_type=Single  exp_bits=8  fraction_bits=24  quantization=Truncate  overflow=Wrap  en=off  latency=1  pipeline=off  dbl_ovrd=off  block_type=convert
  Gateway Out{1..2,4..9,11,13..14} (11 alike) : xbsIndex_r4/Gateway Out  inherit_from_input=off  hdl_port=on  rows=1  columns=1  UseAsDAC=off  DACChannel='1'  interface=None  automatic_assignment=on  address_offset=hex2dec('00')  intf_name=''  intf_description=''  timing_constraint=None  locs_specified=off  LOCs={}  io_standard={}  block_type=gatewayout
  Inverter4 : xbsIndex_r4/Inverter  en=off  latency=1  dbl_ovrd=off  block_type=inv
  Inverter5 : xbsIndex_r4/Inverter  en=off  latency=1  dbl_ovrd=off  block_type=inv
  Register3 : xbsIndex_r4/Register  init=0  rst=on  en=on  dbl_ovrd=off  block_type=register
  Register4 : xbsIndex_r4/Register  init=0  rst=on  en=on  dbl_ovrd=off  block_type=register
  Scope1 : Scope  NumInputPorts=4
  Scope2 : Scope  NumInputPorts=4
  Scope4 : Scope  NumInputPorts=4
  Subsystem : Subsystem
  Subsystem4 : Subsystem
  Subsystem5 : Subsystem
  I_out : Outport
  Q_out : Outport  Port=2
  done : Outport  Port=3
  bit : Outport  Port=4
  wires:
  Accumulator5/1 -> Gateway Out5/1, Register4/1
  Inverter4/1 -> Accumulator4/2
  Inverter5/1 -> Subsystem5/3(Latch), Subsystem4/3(Latch), Accumulator5/2
  Convert10/1 -> Register4/3, Inverter5/1
  Q/1 -> Gateway Out6/1, Accumulator5/1
  Subsystem/3(done) -> done/1
  Register4/1 -> Subsystem5/1(d)
  Window/1 -> Convert10/1, Convert7/1
  I/1 -> Gateway Out8/1, Accumulator4/1
  Reset/1 -> Subsystem5/2(reset), Gateway Out2/1, Subsystem4/2(reset), Register4/2, Register3/2
  Register3/1 -> Subsystem4/1(d)
  Subsystem/4(bit) -> Gateway Out13/1, bit/1
  Subsystem/1(I_norm) -> Gateway Out1/1, I_out/1
  Subsystem/2(Q_norm) -> Gateway Out9/1, Q_out/1
  Gateway Out2/1 -> Scope1/4
  Gateway Out4/1 -> Scope1/1
  Convert7/1 -> Register3/3, Inverter4/1
  Accumulator4/1 -> Gateway Out7/1, Register3/1
  Gateway Out6/1 -> Scope2/3
  Gateway Out5/1 -> Scope2/4
  Gateway Out8/1 -> Scope2/1
  Gateway Out7/1 -> Scope2/2
  Gateway Out1/1 -> Scope1/2
  Subsystem4/1(q) -> Gateway Out11/1, Gateway Out4/1, Subsystem/1(I)
  Subsystem5/1(q) -> Gateway Out14/1, Subsystem/2(Q)
  Gateway Out9/1 -> Scope4/2
  Gateway Out14/1 -> Scope4/1
  Gateway Out11/1 -> Scope4/4
  Gateway Out13/1 -> Scope4/3
